simulink model "second_order_inverse1"  (Simulink 9.2)
settings: Solver=VariableStepAuto  StartTime=0.0  StopTime=4  RelTol=1e-3
undefined symbols (not defined in the file or in its folder): DiscIntNeverNeededParam, q0, q0_dot, Tc
settings Model: Creator=louisling  LastModifiedBy=louisling
settings DataIOCC: LimitDataPoints=off  SaveFormat=Dataset  SignalLoggingSaveFormat=Dataset  ReturnWorkspaceOutputs=on
settings OptimizationCC: LifeSpan=auto
settings DebuggingCC: UnderspecifiedInitializationDetection=Simplified  MergeDetectMultiDrivingBlocksExec=error  FcnCallInpInsideContextMsg=error  StateNameClashWarn=none  SFUnexpectedBacktrackingDiag=error  SFNoUnconditionalDefaultTransitionDiag=error  SFExecutionAtInitializationDiag=warning
settings HardwareCC: ProdBitPerPointer=64  ProdBitPerSizeT=64  ProdBitPerPtrDiffT=64  ProdLargestAtomicFloat=Float  ProdIntDivRoundTo=Zero  ProdEndianess=LittleEndian  ProdWordSize=64  ProdHWDeviceType=Intel->x86-64 (Windows64)
settings ModelReferenceCC: PropagateSignalLabelsOutOfModel=on
settings SFSimCC: SimUseLocalCustomCode=on
settings RTWCC: RTWUseLocalCustomCode=on
settings CodeAppCC: StateflowObjectComments=off
settings GRTTargetCC: TargetLangStandard=C99 (ISO)  GeneratePreprocessorConditionals=Use local settings  CombineOutputUpdateFcns=on  GRTInterface=off
settings ConfigComp: CovMetricSettings=dwe  CovHtmlReporting=off  CovSaveCumulativeToWorkspaceVar=off  CovSaveSingleToWorkspaceVar=off  CovExternalEMLEnable=on

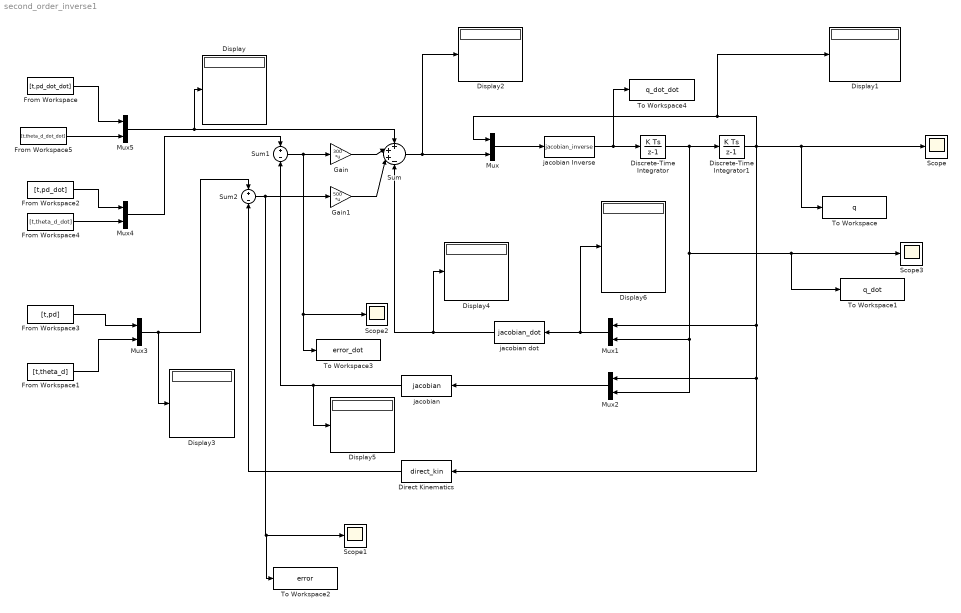
== system second_order_inverse1 ==
  Direct Kinematics : MATLABFcn  MATLABFcn=direct_kin
  Discrete-Time Integrator : DiscreteIntegrator  InitialCondition=q0_dot  SampleTime=Tc  ICPrevOutput=DiscIntNeverNeededParam  ICPrevScaledInput=DiscIntNeverNeededParam
  Discrete-Time Integrator1 : DiscreteIntegrator  InitialCondition=q0  SampleTime=Tc  ICPrevOutput=DiscIntNeverNeededParam  ICPrevScaledInput=DiscIntNeverNeededParam
  Display{,1..6} (7 alike) : Display
  From Workspace : FromWorkspace  VariableName=[t,pd_dot_dot]  SampleTime=0
  From Workspace1 : FromWorkspace  VariableName=[t,theta_d]  SampleTime=0
  From Workspace2 : FromWorkspace  VariableName=[t,pd_dot]  SampleTime=0
  From Workspace3 : FromWorkspace  VariableName=[t,pd]  SampleTime=0
  From Workspace4 : FromWorkspace  VariableName=[t,theta_d_dot]  SampleTime=0
  From Workspace5 : FromWorkspace  VariableName=[t,theta_d_dot_dot]  SampleTime=0
  Gain : Gain  Gain=300  Multiplication=Matrix(K*u)
  Gain1 : Gain  Gain=500  Multiplication=Matrix(K*u)
  Mux{,1..5} (6 alike) : Mux  Inputs=2
  Scope{,1..3} (4 alike) : Scope
  Sum : Sum  Inputs=+++-
  Sum1 : Sum  Inputs=+-
  Sum2 : Sum  Inputs=+-
  To Workspace : ToWorkspace  VariableName=q  SaveFormat=Structure With Time  SampleTime=-1
  To Workspace1 : ToWorkspace  VariableName=q_dot  SaveFormat=Structure With Time  SampleTime=-1
  To Workspace2 : ToWorkspace  VariableName=error  SaveFormat=Structure With Time  SampleTime=-1
  To Workspace3 : ToWorkspace  VariableName=error_dot  SaveFormat=Structure With Time  SampleTime=-1
  To Workspace4 : ToWorkspace  VariableName=q_dot_dot  SaveFormat=Structure With Time  SampleTime=-1
  "jacobian " : MATLABFcn  MATLABFcn=jacobian
  jacobian Inverse : MATLABFcn  MATLABFcn=jacobian_inverse
  jacobian dot : MATLABFcn  MATLABFcn=jacobian_dot
  wires:
  Sum1/1 -> To Workspace3/1, Scope2/1, Gain/1
  Gain/1 -> Sum/2
  "jacobian "/1 -> Display5/1, Sum1/2
  Direct Kinematics/1 -> Sum2/2
  Sum2/1 -> To Workspace2/1, Scope1/1, Gain1/1
  Gain1/1 -> Sum/3
  Discrete-Time Integrator1/1 -> Direct Kinematics/1, Mux2/1, Mux1/1, Mux/1, Display1/1, To Workspace/1, Scope/1
  Mux1/1 -> Display6/1, jacobian dot/1
  jacobian dot/1 -> Display4/1, Sum/4
  Mux2/1 -> "jacobian "/1
  From Workspace1/1 -> Mux3/2
  From Workspace3/1 -> Mux3/1
  Mux3/1 -> Display3/1, Sum2/1
  From Workspace4/1 -> Mux4/2
  From Workspace2/1 -> Mux4/1
  Mux4/1 -> Sum1/1
  From Workspace5/1 -> Mux5/2
  From Workspace/1 -> Mux5/1
  Mux5/1 -> Display/1, Sum/1
  Sum/1 -> Display2/1, Mux/2
  Mux/1 -> jacobian Inverse/1
  jacobian Inverse/1 -> To Workspace4/1, Discrete-Time Integrator/1
  Discrete-Time Integrator/1 -> Mux2/2, Mux1/2, To Workspace1/1, Scope3/1, Discrete-Time Integrator1/1
